simulink model "MyMPCcontroller"  (R2019a)
settings: Solver=VariableStepAuto  StartTime=0.0  StopTime=40  RelTol=1e-3
libraries: simulink x1
settings Model: Creator=neatli  LastModifiedBy=neatli

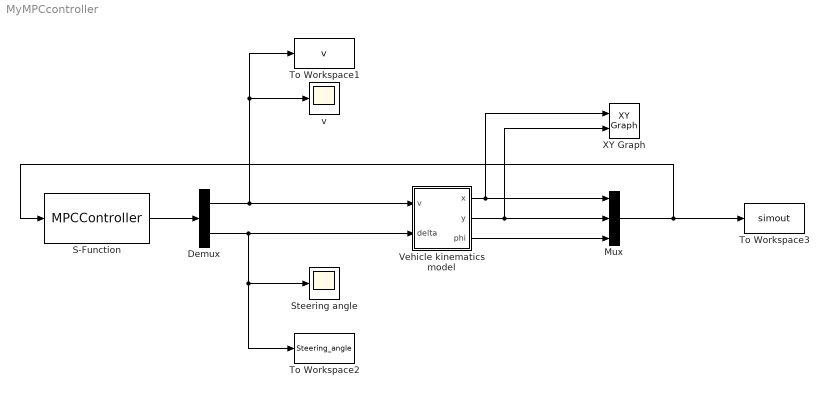
== system MyMPCcontroller ==
  Demux : Demux  Outputs=2
  Mux : Mux  Inputs=3
  S-Function : S-Function  FunctionName=MPCController  SFunctionDeploymentMode=off  EnableBusSupport=off
  Steering angle : Scope
  To Workspace1 : ToWorkspace  VariableName=v  SaveFormat=Timeseries  SampleTime=-1
  To Workspace2 : ToWorkspace  VariableName=Steering_angle  SaveFormat=Timeseries  SampleTime=-1
  To Workspace3 : ToWorkspace  VariableName=simout  SampleTime=-1
  Vehicle kinematics model : Subsystem
  XY Graph : simulink/Sinks/XY Graph  xmin=-30  xmax=30  ymin=-5  ymax=65  st=-1
  v : Scope
  wires:
  Demux/1 -> v/1, To Workspace1/1, Vehicle kinematics model/1(v)
  Demux/2 -> To Workspace2/1, Steering angle/1, Vehicle kinematics model/2(delta)
  Vehicle kinematics model/1(x) -> Mux/1, XY Graph/1
  Vehicle kinematics model/2(y) -> XY Graph/2, Mux/2
  Vehicle kinematics model/3(phi) -> Mux/3
  Mux/1 -> To Workspace3/1, S-Function/1
  S-Function/1 -> Demux/1

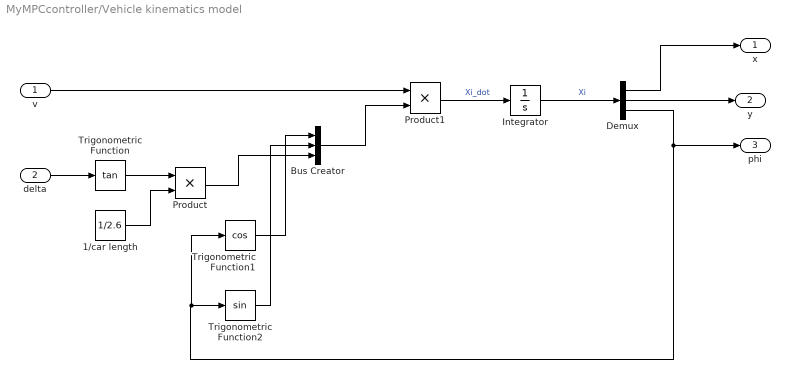
== system MyMPCcontroller/Vehicle kinematics model ==
  v : Inport
  delta : Inport  Port=2
  1/car length : Constant  Value=1/2.6
  Bus Creator : BusCreator  Inputs=3
  Demux : Demux  Outputs=3
  Integrator : Integrator
  Product : Product
  Product1 : Product
  Trigonometric Function : Trigonometry  Operator=tan
  Trigonometric Function1 : Trigonometry  Operator=cos
  Trigonometric Function2 : Trigonometry
  x : Outport
  y : Outport  Port=2
  phi : Outport  Port=3
  wires:
  Product1/1 -> Integrator/1  "Xi_dot"
  v/1 -> Product1/1
  Trigonometric Function1/1 -> Bus Creator/1
  delta/1 -> Trigonometric Function/1
  Trigonometric Function2/1 -> Bus Creator/2
  Demux/1 -> x/1
  Demux/2 -> y/1
  Product/1 -> Bus Creator/3
  1/car length/1 -> Product/2
  Trigonometric Function/1 -> Product/1
  Bus Creator/1 -> Product1/2
  Demux/3 -> phi/1, Trigonometric Function1/1, Trigonometric Function2/1
  Integrator/1 -> Demux/1  "Xi"
